simulink library "inp"  (R2021b)
settings: Solver=VariableStepAuto  StartTime=0.0  StopTime=10.0  RelTol=1e-3
undefined symbols (not defined in the file): C_TASK_5MS_S, FALSE, KINP_AcoreReadyToSlp_flg_ovrdflg, KINP_AcoreReadyToSlp_flg_ovrdval, KINP_AllowMovThd_OTA_enum_ovrdflg, KINP_AllowMovThd_OTA_enum_ovrdval, KINP_APSAngleTarget_Deg_ovrdflg, KINP_APSAngleTarget_Deg_ovrdval, KINP_APSDecReq_mps2_ovrdflg, KINP_APSDecReq_mps2_ovrdval, KINP_APSDecReqA_flg_ovrdflg, KINP_APSDecReqA_flg_ovrdval, KINP_APSDFLL_cm_ovrdflg, KINP_APSDFLL_cm_ovrdval, KINP_APSDFLR_cm_ovrdflg, KINP_APSDFLR_cm_ovrdval, KINP_APSDRLL_cm_ovrdflg, KINP_APSDRLL_cm_ovrdval, KINP_APSDRLR_cm_ovrdflg, KINP_APSDRLR_cm_ovrdval, KINP_APSExitCondition_enum_ovrdflg, KINP_APSExitCondition_enum_ovrdval, KINP_APSHWVer_enum_ovrdflg, KINP_APSHWVer_enum_ovrdval, KINP_APSProgressPCT_pct_ovrdflg, KINP_APSProgressPCT_pct_ovrdval, KINP_APSPwrReq_enum_ovrdflg, KINP_APSPwrReq_enum_ovrdval, KINP_APSReq_enum_ovrdflg, KINP_APSReq_enum_ovrdval, KINP_APSRQDisplay_enum_ovrdflg, KINP_APSRQDisplay_enum_ovrdval, KINP_APSRqEPASCtrl_flg_ovrdflg, KINP_APSRqEPASCtrl_flg_ovrdval, KINP_APSShiftPosnReq_enum_ovrdval, KINP_APSShiftPosnReq_enum_ovrflg, KINP_APSSpeedCMD_kph_ovrdval, KINP_APSSpeedCMD_kph_ovrflg, KINP_APSStaSystem_enum_ovrdflg, KINP_APSStaSystem_enum_ovrdval, KINP_APSSWVer_enum_ovrdflg, KINP_APSSWVer_enum_ovrdval, KINP_APSVMCReqA_flg_ovrdval, KINP_APSVMCReqA_flg_ovrflg, KINP_APSVRqEPASCtrl_flg_ovrdflg, KINP_APSVRqEPASCtrl_flg_ovrdval, KINP_AuxBattVolmV_mV_ovrdflg, KINP_AuxBattVolmV_mV_ovrdval, KINP_BTConnectSta_enum_ovrdflg, KINP_BTConnectSta_enum_ovrdval, KINP_CAASSta_enum_ovrdflg, KINP_CAASSta_enum_ovrdval, KINP_CAASVMCReqA_flg_ovrdval, KINP_CAASVMCReqA_flg_ovrflg, KINP_CAN1BusOff_flg_ovrdflg, KINP_CAN1BusOff_flg_ovrdval, KINP_CAN2BusOff_flg_ovrdflg, KINP_CAN2BusOff_flg_ovrdval, KINP_CAN3BusOff_flg_ovrdflg, KINP_CAN3BusOff_flg_ovrdval ... (+222)
libraries: FVT_lib x1035, hcu_lib x1
(part 24 of 33)

== system inp/INP/CAN3/SignalCheck/MCU_N_F2 ==
  BHAL_outputs : Inport
  inp_CanValid_bus : Inport  Port=2
  FrCoolanttempReqNidec : FVT_lib/inp/can_signal_template  SystemSampleTime=-1  VariantActivationTime=update diagram  Latency=0  AutoFrameSizeCalculation=off
      link override defval: Value=KINP_FrCoolanttempReqNidec_C_defval
      link override ovrdflg: Value=KINP_FrCoolanttempReqNidec_C_ovrdflg
      link override ovrdval: Value=KINP_FrCoolanttempReqNidec_C_ovrdval
  FrEOPSpdSetNidec : FVT_lib/inp/can_signal_template  SystemSampleTime=-1  VariantActivationTime=update diagram  Latency=0  AutoFrameSizeCalculation=off
      link override defval: Value=KINP_FrEOPSpdSetNidec_rpm_defval
      link override ovrdflg: Value=KINP_FrEOPSpdSetNidec_rpm_ovrdflg
      link override ovrdval: Value=KINP_FrEOPSpdSetNidec_rpm_ovrdval
  FrFailcode1Nidec : FVT_lib/inp/can_signal_template  SystemSampleTime=-1  VariantActivationTime=update diagram  Latency=0  AutoFrameSizeCalculation=off
      link override defval: Value=KINP_FrFailcode1Nidec_enum_defval
      link override ovrdflg: Value=KINP_FrFailcode1Nidec_enum_ovrdflg
      link override ovrdval: Value=KINP_FrFailcode1Nidec_enum_ovrdval
  FrFailcode2Nidec : FVT_lib/inp/can_signal_template  SystemSampleTime=-1  VariantActivationTime=update diagram  Latency=0  AutoFrameSizeCalculation=off
      link override defval: Value=KINP_FrFailcode2Nidec_enum_defval
      link override ovrdflg: Value=KINP_FrFailcode2Nidec_enum_ovrdflg
      link override ovrdval: Value=KINP_FrFailcode2Nidec_enum_ovrdval
  FrFailcodehistory1Nidec : FVT_lib/inp/can_signal_template  SystemSampleTime=-1  VariantActivationTime=update diagram  Latency=0  AutoFrameSizeCalculation=off
      link override defval: Value=KINP_FrFailcodehistory1Nidec_enum_defval
      link override ovrdflg: Value=KINP_FrFailcodehistory1Nidec_enum_ovrdflg
      link override ovrdval: Value=KINP_FrFailcodehistory1Nidec_enum_ovrdval
  FrFailcodehistory2Nidec : FVT_lib/inp/can_signal_template  SystemSampleTime=-1  VariantActivationTime=update diagram  Latency=0  AutoFrameSizeCalculation=off
      link override defval: Value=KINP_FrFailcodehistory2Nidec_enum_defval
      link override ovrdflg: Value=KINP_FrFailcodehistory2Nidec_enum_ovrdflg
      link override ovrdval: Value=KINP_FrFailcodehistory2Nidec_enum_ovrdval
  FrLLCTempNidec : FVT_lib/inp/can_signal_template  SystemSampleTime=-1  VariantActivationTime=update diagram  Latency=0  AutoFrameSizeCalculation=off
      link override defval: Value=KINP_FrLLCTempNidec_C_defval
      link override ovrdflg: Value=KINP_FrLLCTempNidec_C_ovrdflg
      link override ovrdval: Value=KINP_FrLLCTempNidec_C_ovrdval
  FrLLCflowReqNidec : FVT_lib/inp/can_signal_template  SystemSampleTime=-1  VariantActivationTime=update diagram  Latency=0  AutoFrameSizeCalculation=off
      link override defval: Value=KINP_FrLLCflowReqNidec_Lpmin_defval
      link override ovrdflg: Value=KINP_FrLLCflowReqNidec_Lpmin_ovrdflg
      link override ovrdval: Value=KINP_FrLLCflowReqNidec_Lpmin_ovrdval
  FrMCUTempWarnNidec : FVT_lib/inp/can_signal_template  SystemSampleTime=-1  VariantActivationTime=update diagram  Latency=0  AutoFrameSizeCalculation=off
      link override defval: Value=KINP_FrMCUTempWarnNidec_enum_defval
      link override ovrdflg: Value=KINP_FrMCUTempWarnNidec_enum_ovrdflg
      link override ovrdval: Value=KINP_FrMCUTempWarnNidec_enum_ovrdval
  FrTMTempWarnNidec : FVT_lib/inp/can_signal_template  SystemSampleTime=-1  VariantActivationTime=update diagram  Latency=0  AutoFrameSizeCalculation=off
      link override defval: Value=KINP_FrTMTempWarnNidec_enum_defval
      link override ovrdflg: Value=KINP_FrTMTempWarnNidec_enum_ovrdflg
      link override ovrdval: Value=KINP_FrTMTempWarnNidec_enum_ovrdval
  Terminator_{1..10} (10 alike) : Terminator
  True_VHAL_FrCoolanttempReqNidec_C : Constant  Value=TRUE  OutDataTypeStr=boolean
  True_VHAL_FrEOPSpdSetNidec_rpm : Constant  Value=TRUE  OutDataTypeStr=boolean
  True_VHAL_FrFailcode1Nidec_enum : Constant  Value=TRUE  OutDataTypeStr=boolean
  True_VHAL_FrFailcode2Nidec_enum : Constant  Value=TRUE  OutDataTypeStr=boolean
  True_VHAL_FrFailcodehistory1Nidec_enum : Constant  Value=TRUE  OutDataTypeStr=boolean
  True_VHAL_FrFailcodehistory2Nidec_enum : Constant  Value=TRUE  OutDataTypeStr=boolean
  True_VHAL_FrLLCTempNidec_C : Constant  Value=TRUE  OutDataTypeStr=boolean
  True_VHAL_FrLLCflowReqNidec_Lpmin : Constant  Value=TRUE  OutDataTypeStr=boolean
  True_VHAL_FrMCUTempWarnNidec_enum : Constant  Value=TRUE  OutDataTypeStr=boolean
  True_VHAL_FrTMTempWarnNidec_enum : Constant  Value=TRUE  OutDataTypeStr=boolean
  slr1_{1..10} (10 alike) : BusSelector  OutputSignals=VINP_CANMsgValidMCUNF2_flg
  slr_VHAL_FrCoolanttempReqNidec_C : BusSelector  OutputSignals=VHAL_FrCoolanttempReqNidec_C
  slr_VHAL_FrEOPSpdSetNidec_rpm : BusSelector  OutputSignals=VHAL_FrEOPSpdSetNidec_rpm
  slr_VHAL_FrFailcode1Nidec_enum : BusSelector  OutputSignals=VHAL_FrFailcode1Nidec_enum
  slr_VHAL_FrFailcode2Nidec_enum : BusSelector  OutputSignals=VHAL_FrFailcode2Nidec_enum
  slr_VHAL_FrFailcodehistory1Nidec_enum : BusSelector  OutputSignals=VHAL_FrFailcodehistory1Nidec_enum
  slr_VHAL_FrFailcodehistory2Nidec_enum : BusSelector  OutputSignals=VHAL_FrFailcodehistory2Nidec_enum
  slr_VHAL_FrLLCTempNidec_C : BusSelector  OutputSignals=VHAL_FrLLCTempNidec_C
  slr_VHAL_FrLLCflowReqNidec_Lpmin : BusSelector  OutputSignals=VHAL_FrLLCflowReqNidec_Lpmin
  slr_VHAL_FrMCUTempWarnNidec_enum : BusSelector  OutputSignals=VHAL_FrMCUTempWarnNidec_enum
  slr_VHAL_FrTMTempWarnNidec_enum : BusSelector  OutputSignals=VHAL_FrTMTempWarnNidec_enum
  VINP_FrCoolanttempReqNidec_C : Outport
  VINP_FrEOPSpdSetNidec_rpm : Outport  Port=2
  VINP_FrFailcode1Nidec_enum : Outport  Port=3
  VINP_FrFailcode2Nidec_enum : Outport  Port=4
  VINP_FrFailcodehistory1Nidec_enum : Outport  Port=5
  VINP_FrFailcodehistory2Nidec_enum : Outport  Port=6
  VINP_FrLLCTempNidec_C : Outport  Port=7
  VINP_FrLLCflowReqNidec_Lpmin : Outport  Port=8
  VINP_FrMCUTempWarnNidec_enum : Outport  Port=9
  VINP_FrTMTempWarnNidec_enum : Outport  Port=10
  wires:
  BHAL_outputs/1 -> [BHAL_outputs]
  inp_CanValid_bus/1 -> [inp_CanValid_bus]
  [BHAL_outputs] -> slr_VHAL_FrCoolanttempReqNidec_C/1
  slr_VHAL_FrCoolanttempReqNidec_C/1 -> FrCoolanttempReqNidec/1  "<VHAL_FrCoolanttempReqNidec_C>"
  True_VHAL_FrCoolanttempReqNidec_C/1 -> FrCoolanttempReqNidec/2
  [inp_CanValid_bus] -> slr1_1/1
  slr1_1/1 -> FrCoolanttempReqNidec/3  "<VINP_CANMsgValidMCUNF2_flg>"
  FrCoolanttempReqNidec/1 -> VINP_FrCoolanttempReqNidec_C/1  "VINP_FrCoolanttempReqNidec_C"
  FrCoolanttempReqNidec/2 -> Terminator_1/1
  [BHAL_outputs] -> slr_VHAL_FrEOPSpdSetNidec_rpm/1
  slr_VHAL_FrEOPSpdSetNidec_rpm/1 -> FrEOPSpdSetNidec/1  "<VHAL_FrEOPSpdSetNidec_rpm>"
  True_VHAL_FrEOPSpdSetNidec_rpm/1 -> FrEOPSpdSetNidec/2
  [inp_CanValid_bus] -> slr1_2/1
  slr1_2/1 -> FrEOPSpdSetNidec/3  "<VINP_CANMsgValidMCUNF2_flg>"
  FrEOPSpdSetNidec/1 -> VINP_FrEOPSpdSetNidec_rpm/1  "VINP_FrEOPSpdSetNidec_rpm"
  FrEOPSpdSetNidec/2 -> Terminator_2/1
  [BHAL_outputs] -> slr_VHAL_FrFailcode1Nidec_enum/1
  slr_VHAL_FrFailcode1Nidec_enum/1 -> FrFailcode1Nidec/1  "<VHAL_FrFailcode1Nidec_enum>"
  True_VHAL_FrFailcode1Nidec_enum/1 -> FrFailcode1Nidec/2
  [inp_CanValid_bus] -> slr1_3/1
  slr1_3/1 -> FrFailcode1Nidec/3  "<VINP_CANMsgValidMCUNF2_flg>"
  FrFailcode1Nidec/1 -> VINP_FrFailcode1Nidec_enum/1  "VINP_FrFailcode1Nidec_enum"
  FrFailcode1Nidec/2 -> Terminator_3/1
  [BHAL_outputs] -> slr_VHAL_FrFailcode2Nidec_enum/1
  slr_VHAL_FrFailcode2Nidec_enum/1 -> FrFailcode2Nidec/1  "<VHAL_FrFailcode2Nidec_enum>"
  True_VHAL_FrFailcode2Nidec_enum/1 -> FrFailcode2Nidec/2
  [inp_CanValid_bus] -> slr1_4/1
  slr1_4/1 -> FrFailcode2Nidec/3  "<VINP_CANMsgValidMCUNF2_flg>"
  FrFailcode2Nidec/1 -> VINP_FrFailcode2Nidec_enum/1  "VINP_FrFailcode2Nidec_enum"
  FrFailcode2Nidec/2 -> Terminator_4/1
  [BHAL_outputs] -> slr_VHAL_FrFailcodehistory1Nidec_enum/1
  slr_VHAL_FrFailcodehistory1Nidec_enum/1 -> FrFailcodehistory1Nidec/1  "<VHAL_FrFailcodehistory1Nidec_enum>"
  True_VHAL_FrFailcodehistory1Nidec_enum/1 -> FrFailcodehistory1Nidec/2
  [inp_CanValid_bus] -> slr1_5/1
  slr1_5/1 -> FrFailcodehistory1Nidec/3  "<VINP_CANMsgValidMCUNF2_flg>"
  FrFailcodehistory1Nidec/1 -> VINP_FrFailcodehistory1Nidec_enum/1  "VINP_FrFailcodehistory1Nidec_enum"
  FrFailcodehistory1Nidec/2 -> Terminator_5/1
  [BHAL_outputs] -> slr_VHAL_FrFailcodehistory2Nidec_enum/1
  slr_VHAL_FrFailcodehistory2Nidec_enum/1 -> FrFailcodehistory2Nidec/1  "<VHAL_FrFailcodehistory2Nidec_enum>"
  True_VHAL_FrFailcodehistory2Nidec_enum/1 -> FrFailcodehistory2Nidec/2
  [inp_CanValid_bus] -> slr1_6/1
  slr1_6/1 -> FrFailcodehistory2Nidec/3  "<VINP_CANMsgValidMCUNF2_flg>"
  FrFailcodehistory2Nidec/1 -> VINP_FrFailcodehistory2Nidec_enum/1  "VINP_FrFailcodehistory2Nidec_enum"
  FrFailcodehistory2Nidec/2 -> Terminator_6/1
  [BHAL_outputs] -> slr_VHAL_FrLLCTempNidec_C/1
  slr_VHAL_FrLLCTempNidec_C/1 -> FrLLCTempNidec/1  "<VHAL_FrLLCTempNidec_C>"
  True_VHAL_FrLLCTempNidec_C/1 -> FrLLCTempNidec/2
  [inp_CanValid_bus] -> slr1_7/1
  slr1_7/1 -> FrLLCTempNidec/3  "<VINP_CANMsgValidMCUNF2_flg>"
  FrLLCTempNidec/1 -> VINP_FrLLCTempNidec_C/1  "VINP_FrLLCTempNidec_C"
  FrLLCTempNidec/2 -> Terminator_7/1
  [BHAL_outputs] -> slr_VHAL_FrLLCflowReqNidec_Lpmin/1
  slr_VHAL_FrLLCflowReqNidec_Lpmin/1 -> FrLLCflowReqNidec/1  "<VHAL_FrLLCflowReqNidec_Lpmin>"
  True_VHAL_FrLLCflowReqNidec_Lpmin/1 -> FrLLCflowReqNidec/2
  [inp_CanValid_bus] -> slr1_8/1
  slr1_8/1 -> FrLLCflowReqNidec/3  "<VINP_CANMsgValidMCUNF2_flg>"
  FrLLCflowReqNidec/1 -> VINP_FrLLCflowReqNidec_Lpmin/1  "VINP_FrLLCflowReqNidec_Lpmin"
  FrLLCflowReqNidec/2 -> Terminator_8/1
  [BHAL_outputs] -> slr_VHAL_FrMCUTempWarnNidec_enum/1
  slr_VHAL_FrMCUTempWarnNidec_enum/1 -> FrMCUTempWarnNidec/1  "<VHAL_FrMCUTempWarnNidec_enum>"
  True_VHAL_FrMCUTempWarnNidec_enum/1 -> FrMCUTempWarnNidec/2
  [inp_CanValid_bus] -> slr1_9/1
  slr1_9/1 -> FrMCUTempWarnNidec/3  "<VINP_CANMsgValidMCUNF2_flg>"
  FrMCUTempWarnNidec/1 -> VINP_FrMCUTempWarnNidec_enum/1  "VINP_FrMCUTempWarnNidec_enum"
  FrMCUTempWarnNidec/2 -> Terminator_9/1
  [BHAL_outputs] -> slr_VHAL_FrTMTempWarnNidec_enum/1
  slr_VHAL_FrTMTempWarnNidec_enum/1 -> FrTMTempWarnNidec/1  "<VHAL_FrTMTempWarnNidec_enum>"
  True_VHAL_FrTMTempWarnNidec_enum/1 -> FrTMTempWarnNidec/2
  [inp_CanValid_bus] -> slr1_10/1
  slr1_10/1 -> FrTMTempWarnNidec/3  "<VINP_CANMsgValidMCUNF2_flg>"
  FrTMTempWarnNidec/1 -> VINP_FrTMTempWarnNidec_enum/1  "VINP_FrTMTempWarnNidec_enum"
  FrTMTempWarnNidec/2 -> Terminator_10/1

== system inp/INP/CAN3/SignalCheck/MCU_N_F3 ==
  BHAL_outputs : Inport
  inp_CanValid_bus : Inport  Port=2
  FrMCUHWVerNidec : FVT_lib/inp/can_signal_template  SystemSampleTime=-1  VariantActivationTime=update diagram  Latency=0  AutoFrameSizeCalculation=off
      link override defval: Value=KINP_FrMCUHWVerNidec_enum_defval
      link override ovrdflg: Value=KINP_FrMCUHWVerNidec_enum_ovrdflg
      link override ovrdval: Value=KINP_FrMCUHWVerNidec_enum_ovrdval
  FrMCUSWVerNidec : FVT_lib/inp/can_signal_template  SystemSampleTime=-1  VariantActivationTime=update diagram  Latency=0  AutoFrameSizeCalculation=off
      link override defval: Value=KINP_FrMCUSWVerNidec_enum_defval
      link override ovrdflg: Value=KINP_FrMCUSWVerNidec_enum_ovrdflg
      link override ovrdval: Value=KINP_FrMCUSWVerNidec_enum_ovrdval
  Terminator_1 : Terminator
  Terminator_2 : Terminator
  True_VHAL_FrMCUHWVerNidec_enum : Constant  Value=TRUE  OutDataTypeStr=boolean
  True_VHAL_FrMCUSWVerNidec_enum : Constant  Value=TRUE  OutDataTypeStr=boolean
  slr1_1 : BusSelector  OutputSignals=VINP_CANMsgValidMCUNF3_flg
  slr1_2 : BusSelector  OutputSignals=VINP_CANMsgValidMCUNF3_flg
  slr_VHAL_FrMCUHWVerNidec_enum : BusSelector  OutputSignals=VHAL_FrMCUHWVerNidec_enum
  slr_VHAL_FrMCUSWVerNidec_enum : BusSelector  OutputSignals=VHAL_FrMCUSWVerNidec_enum
  VINP_FrMCUHWVerNidec_enum : Outport
  VINP_FrMCUSWVerNidec_enum : Outport  Port=2
  wires:
  BHAL_outputs/1 -> [BHAL_outputs]
  inp_CanValid_bus/1 -> [inp_CanValid_bus]
  [BHAL_outputs] -> slr_VHAL_FrMCUHWVerNidec_enum/1
  slr_VHAL_FrMCUHWVerNidec_enum/1 -> FrMCUHWVerNidec/1  "<VHAL_FrMCUHWVerNidec_enum>"
  True_VHAL_FrMCUHWVerNidec_enum/1 -> FrMCUHWVerNidec/2
  [inp_CanValid_bus] -> slr1_1/1
  slr1_1/1 -> FrMCUHWVerNidec/3  "<VINP_CANMsgValidMCUNF3_flg>"
  FrMCUHWVerNidec/1 -> VINP_FrMCUHWVerNidec_enum/1  "VINP_FrMCUHWVerNidec_enum"
  FrMCUHWVerNidec/2 -> Terminator_1/1
  [BHAL_outputs] -> slr_VHAL_FrMCUSWVerNidec_enum/1
  slr_VHAL_FrMCUSWVerNidec_enum/1 -> FrMCUSWVerNidec/1  "<VHAL_FrMCUSWVerNidec_enum>"
  True_VHAL_FrMCUSWVerNidec_enum/1 -> FrMCUSWVerNidec/2
  [inp_CanValid_bus] -> slr1_2/1
  slr1_2/1 -> FrMCUSWVerNidec/3  "<VINP_CANMsgValidMCUNF3_flg>"
  FrMCUSWVerNidec/1 -> VINP_FrMCUSWVerNidec_enum/1  "VINP_FrMCUSWVerNidec_enum"
  FrMCUSWVerNidec/2 -> Terminator_2/1

== system inp/INP/CAN3/SignalCheck/MCU_N_R1 ==
  BHAL_outputs : Inport
  inp_CanValid_bus : Inport  Port=2
  MCUNR1CSErr : FVT_lib/inp/can_signal_template  SystemSampleTime=-1  VariantActivationTime=update diagram  Latency=0  AutoFrameSizeCalculation=off
      link override defval: Value=KINP_MCUNR1CSErr_flg_defval
      link override ovrdflg: Value=KINP_MCUNR1CSErr_flg_ovrdflg
      link override ovrdval: Value=KINP_MCUNR1CSErr_flg_ovrdval
  MCUNR1RCErr : FVT_lib/inp/can_signal_template  SystemSampleTime=-1  VariantActivationTime=update diagram  Latency=0  AutoFrameSizeCalculation=off
      link override defval: Value=KINP_MCUNR1RCErr_flg_defval
      link override ovrdflg: Value=KINP_MCUNR1RCErr_flg_ovrdflg
      link override ovrdval: Value=KINP_MCUNR1RCErr_flg_ovrdval
  MCUWarnRNidec : FVT_lib/inp/can_signal_template  SystemSampleTime=-1  VariantActivationTime=update diagram  Latency=0  AutoFrameSizeCalculation=off
      link override defval: Value=KINP_MCUWarnRNidec_enum_defval
      link override ovrdflg: Value=KINP_MCUWarnRNidec_enum_ovrdflg
      link override ovrdval: Value=KINP_MCUWarnRNidec_enum_ovrdval
  RrActvDmpDisabStaNidec : FVT_lib/inp/can_signal_template  SystemSampleTime=-1  VariantActivationTime=update diagram  Latency=0  AutoFrameSizeCalculation=off
      link override defval: Value=KINP_RrActvDmpDisabStaNidec_flg_defval
      link override ovrdflg: Value=KINP_RrActvDmpDisabStaNidec_flg_ovrdflg
      link override ovrdval: Value=KINP_RrActvDmpDisabStaNidec_flg_ovrdval
  RrEDUDrtStaNidec : FVT_lib/inp/can_signal_template  SystemSampleTime=-1  VariantActivationTime=update diagram  Latency=0  AutoFrameSizeCalculation=off
      link override defval: Value=KINP_RrEDUDrtStaNidec_flg_defval
      link override ovrdflg: Value=KINP_RrEDUDrtStaNidec_flg_ovrdflg
      link override ovrdval: Value=KINP_RrEDUDrtStaNidec_flg_ovrdval
  RrEDUOpratingStaNidec : FVT_lib/inp/can_signal_template  SystemSampleTime=-1  VariantActivationTime=update diagram  Latency=0  AutoFrameSizeCalculation=off
      link override defval: Value=KINP_RrEDUOpratingStaNidec_flg_defval
      link override ovrdflg: Value=KINP_RrEDUOpratingStaNidec_flg_ovrdflg
      link override ovrdval: Value=KINP_RrEDUOpratingStaNidec_flg_ovrdval
  RrEDURealTMTqNidec : FVT_lib/inp/can_signal_template  SystemSampleTime=-1  VariantActivationTime=update diagram  Latency=0  AutoFrameSizeCalculation=off
      link override defval: Value=KINP_RrEDURealTMTqNidec_Nm_defval
      link override ovrdflg: Value=KINP_RrEDURealTMTqNidec_Nm_ovrdflg
      link override ovrdval: Value=KINP_RrEDURealTMTqNidec_Nm_ovrdval
  RrEDURotateDirctionNidec : FVT_lib/inp/can_signal_template  SystemSampleTime=-1  VariantActivationTime=update diagram  Latency=0  AutoFrameSizeCalculation=off
      link override defval: Value=KINP_RrEDURotateDirctionNidec_enum_defval
      link override ovrdflg: Value=KINP_RrEDURotateDirctionNidec_enum_ovrdflg
      link override ovrdval: Value=KINP_RrEDURotateDirctionNidec_enum_ovrdval
  RrEDUTqReqFbkNidec : FVT_lib/inp/can_signal_template  SystemSampleTime=-1  VariantActivationTime=update diagram  Latency=0  AutoFrameSizeCalculation=off
      link override defval: Value=KINP_RrEDUTqReqFbkNidec_Nm_defval
      link override ovrdflg: Value=KINP_RrEDUTqReqFbkNidec_Nm_ovrdflg
      link override ovrdval: Value=KINP_RrEDUTqReqFbkNidec_Nm_ovrdval
  RrMCU1ChksumNidec : FVT_lib/inp/can_signal_template  SystemSampleTime=-1  VariantActivationTime=update diagram  Latency=0  AutoFrameSizeCalculation=off
      link override defval: Value=KINP_RrMCU1ChksumNidec_enum_defval
      link override ovrdflg: Value=KINP_RrMCU1ChksumNidec_enum_ovrdflg
      link override ovrdval: Value=KINP_RrMCU1ChksumNidec_enum_ovrdval
  RrMCU1RolCntNidec : FVT_lib/inp/can_signal_template  SystemSampleTime=-1  VariantActivationTime=update diagram  Latency=0  AutoFrameSizeCalculation=off
      link override defval: Value=KINP_RrMCU1RolCntNidec_enum_defval
      link override ovrdflg: Value=KINP_RrMCU1RolCntNidec_enum_ovrdflg
      link override ovrdval: Value=KINP_RrMCU1RolCntNidec_enum_ovrdval
  RrMCUBATNidec : FVT_lib/inp/can_signal_template  SystemSampleTime=-1  VariantActivationTime=update diagram  Latency=0  AutoFrameSizeCalculation=off
      link override defval: Value=KINP_RrMCUBATNidec_V_defval
      link override ovrdflg: Value=KINP_RrMCUBATNidec_V_ovrdflg
      link override ovrdval: Value=KINP_RrMCUBATNidec_V_ovrdval
  RrMCUDCBusCurrNidec : FVT_lib/inp/can_signal_template  SystemSampleTime=-1  VariantActivationTime=update diagram  Latency=0  AutoFrameSizeCalculation=off
      link override defval: Value=KINP_RrMCUDCBusCurrNidec_A_defval
      link override ovrdflg: Value=KINP_RrMCUDCBusCurrNidec_A_ovrdflg
      link override ovrdval: Value=KINP_RrMCUDCBusCurrNidec_A_ovrdval
  RrMCUDCBusVoltNidec : FVT_lib/inp/can_signal_template  SystemSampleTime=-1  VariantActivationTime=update diagram  Latency=0  AutoFrameSizeCalculation=off
      link override defval: Value=KINP_RrMCUDCBusVoltNidec_V_defval
      link override ovrdflg: Value=KINP_RrMCUDCBusVoltNidec_V_ovrdflg
      link override ovrdval: Value=KINP_RrMCUDCBusVoltNidec_V_ovrdval
  RrMCUDischrgStaNidec : FVT_lib/inp/can_signal_template  SystemSampleTime=-1  VariantActivationTime=update diagram  Latency=0  AutoFrameSizeCalculation=off
      link override defval: Value=KINP_RrMCUDischrgStaNidec_flg_defval
      link override ovrdflg: Value=KINP_RrMCUDischrgStaNidec_flg_ovrdflg
      link override ovrdval: Value=KINP_RrMCUDischrgStaNidec_flg_ovrdval
  RrMCUEnaStaNidec : FVT_lib/inp/can_signal_template  SystemSampleTime=-1  VariantActivationTime=update diagram  Latency=0  AutoFrameSizeCalculation=off
      link override defval: Value=KINP_RrMCUEnaStaNidec_flg_defval
      link override ovrdflg: Value=KINP_RrMCUEnaStaNidec_flg_ovrdflg
      link override ovrdval: Value=KINP_RrMCUEnaStaNidec_flg_ovrdval
  RrMCUErrNidec : FVT_lib/inp/can_signal_template  SystemSampleTime=-1  VariantActivationTime=update diagram  Latency=0  AutoFrameSizeCalculation=off
      link override defval: Value=KINP_RrMCUErrNidec_enum_defval
      link override ovrdflg: Value=KINP_RrMCUErrNidec_enum_ovrdflg
      link override ovrdval: Value=KINP_RrMCUErrNidec_enum_ovrdval
  RrMCUIGNstaNidec : FVT_lib/inp/can_signal_template  SystemSampleTime=-1  VariantActivationTime=update diagram  Latency=0  AutoFrameSizeCalculation=off
      link override defval: Value=KINP_RrMCUIGNstaNidec_flg_defval
      link override ovrdflg: Value=KINP_RrMCUIGNstaNidec_flg_ovrdflg
      link override ovrdval: Value=KINP_RrMCUIGNstaNidec_flg_ovrdval
  RrMCUReady4PreNidec : FVT_lib/inp/can_signal_template  SystemSampleTime=-1  VariantActivationTime=update diagram  Latency=0  AutoFrameSizeCalculation=off
      link override defval: Value=KINP_RrMCUReady4PreNidec_flg_defval
      link override ovrdflg: Value=KINP_RrMCUReady4PreNidec_flg_ovrdflg
      link override ovrdval: Value=KINP_RrMCUReady4PreNidec_flg_ovrdval
  RrMCUReadyNidec : FVT_lib/inp/can_signal_template  SystemSampleTime=-1  VariantActivationTime=update diagram  Latency=0  AutoFrameSizeCalculation=off
      link override defval: Value=KINP_RrMCUReadyNidec_flg_defval
      link override ovrdflg: Value=KINP_RrMCUReadyNidec_flg_ovrdflg
      link override ovrdval: Value=KINP_RrMCUReadyNidec_flg_ovrdval
  RrMCUSysStaNidec : FVT_lib/inp/can_signal_template  SystemSampleTime=-1  VariantActivationTime=update diagram  Latency=0  AutoFrameSizeCalculation=off
      link override defval: Value=KINP_RrMCUSysStaNidec_enum_defval
      link override ovrdflg: Value=KINP_RrMCUSysStaNidec_enum_ovrdflg
      link override ovrdval: Value=KINP_RrMCUSysStaNidec_enum_ovrdval
  RrMCUTempNidec : FVT_lib/inp/can_signal_template  SystemSampleTime=-1  VariantActivationTime=update diagram  Latency=0  AutoFrameSizeCalculation=off
      link override defval: Value=KINP_RrMCUTempNidec_C_defval
      link override ovrdflg: Value=KINP_RrMCUTempNidec_C_ovrdflg
      link override ovrdval: Value=KINP_RrMCUTempNidec_C_ovrdval
  RrMotorAvailTqNidec : FVT_lib/inp/can_signal_template  SystemSampleTime=-1  VariantActivationTime=update diagram  Latency=0  AutoFrameSizeCalculation=off
      link override defval: Value=KINP_RrMotorAvailTqNidec_Nm_defval
      link override ovrdflg: Value=KINP_RrMotorAvailTqNidec_Nm_ovrdflg
      link override ovrdval: Value=KINP_RrMotorAvailTqNidec_Nm_ovrdval
  RrRegenAvailTqNidec : FVT_lib/inp/can_signal_template  SystemSampleTime=-1  VariantActivationTime=update diagram  Latency=0  AutoFrameSizeCalculation=off
      link override defval: Value=KINP_RrRegenAvailTqNidec_Nm_defval
      link override ovrdflg: Value=KINP_RrRegenAvailTqNidec_Nm_ovrdflg
      link override ovrdval: Value=KINP_RrRegenAvailTqNidec_Nm_ovrdval
  RrTMSpdNidec : FVT_lib/inp/can_signal_template  SystemSampleTime=-1  VariantActivationTime=update diagram  Latency=0  AutoFrameSizeCalculation=off
      link override defval: Value=KINP_RrTMSpdNidec_rpm_defval
      link override ovrdflg: Value=KINP_RrTMSpdNidec_rpm_ovrdflg
      link override ovrdval: Value=KINP_RrTMSpdNidec_rpm_ovrdval
  RrTMTempNidec : FVT_lib/inp/can_signal_template  SystemSampleTime=-1  VariantActivationTime=update diagram  Latency=0  AutoFrameSizeCalculation=off
      link override defval: Value=KINP_RrTMTempNidec_C_defval
      link override ovrdflg: Value=KINP_RrTMTempNidec_C_ovrdflg
      link override ovrdval: Value=KINP_RrTMTempNidec_C_ovrdval
  RrTMidNidec : FVT_lib/inp/can_signal_template  SystemSampleTime=-1  VariantActivationTime=update diagram  Latency=0  AutoFrameSizeCalculation=off
      link override defval: Value=KINP_RrTMidNidec_A_defval
      link override ovrdflg: Value=KINP_RrTMidNidec_A_ovrdflg
      link override ovrdval: Value=KINP_RrTMidNidec_A_ovrdval
  RrTMiqNidec : FVT_lib/inp/can_signal_template  SystemSampleTime=-1  VariantActivationTime=update diagram  Latency=0  AutoFrameSizeCalculation=off
      link override defval: Value=KINP_RrTMiqNidec_A_defval
      link override ovrdflg: Value=KINP_RrTMiqNidec_A_ovrdflg
      link override ovrdval: Value=KINP_RrTMiqNidec_A_ovrdval
  Terminator_{1..28} (28 alike) : Terminator
  True_VHAL_MCUNR1CSErr_flg : Constant  Value=TRUE  OutDataTypeStr=boolean
  True_VHAL_MCUNR1RCErr_flg : Constant  Value=TRUE  OutDataTypeStr=boolean
  True_VHAL_MCUWarnRNidec_enum : Constant  Value=TRUE  OutDataTypeStr=boolean
  True_VHAL_RrActvDmpDisabStaNidec_flg : Constant  Value=TRUE  OutDataTypeStr=boolean
  True_VHAL_RrEDUDrtStaNidec_flg : Constant  Value=TRUE  OutDataTypeStr=boolean
  True_VHAL_RrEDUOpratingStaNidec_flg : Constant  Value=TRUE  OutDataTypeStr=boolean
  True_VHAL_RrEDURealTMTqNidec_Nm : Constant  Value=TRUE  OutDataTypeStr=boolean
  True_VHAL_RrEDURotateDirctionNidec_enum : Constant  Value=TRUE  OutDataTypeStr=boolean
  True_VHAL_RrEDUTqReqFbkNidec_Nm : Constant  Value=TRUE  OutDataTypeStr=boolean
  True_VHAL_RrMCU1ChksumNidec_enum : Constant  Value=TRUE  OutDataTypeStr=boolean
  True_VHAL_RrMCU1RolCntNidec_enum : Constant  Value=TRUE  OutDataTypeStr=boolean
  True_VHAL_RrMCUBATNidec_V : Constant  Value=TRUE  OutDataTypeStr=boolean
  True_VHAL_RrMCUDCBusCurrNidec_A : Constant  Value=TRUE  OutDataTypeStr=boolean
  True_VHAL_RrMCUDCBusVoltNidec_V : Constant  Value=TRUE  OutDataTypeStr=boolean
  True_VHAL_RrMCUDischrgStaNidec_flg : Constant  Value=TRUE  OutDataTypeStr=boolean
  True_VHAL_RrMCUEnaStaNidec_flg : Constant  Value=TRUE  OutDataTypeStr=boolean
  True_VHAL_RrMCUErrNidec_enum : Constant  Value=TRUE  OutDataTypeStr=boolean
  True_VHAL_RrMCUIGNstaNidec_flg : Constant  Value=TRUE  OutDataTypeStr=boolean
  True_VHAL_RrMCUReady4PreNidec_flg : Constant  Value=TRUE  OutDataTypeStr=boolean
  True_VHAL_RrMCUReadyNidec_flg : Constant  Value=TRUE  OutDataTypeStr=boolean
  True_VHAL_RrMCUSysStaNidec_enum : Constant  Value=TRUE  OutDataTypeStr=boolean
  True_VHAL_RrMCUTempNidec_C : Constant  Value=TRUE  OutDataTypeStr=boolean
  True_VHAL_RrMotorAvailTqNidec_Nm : Constant  Value=TRUE  OutDataTypeStr=boolean
  True_VHAL_RrRegenAvailTqNidec_Nm : Constant  Value=TRUE  OutDataTypeStr=boolean
  True_VHAL_RrTMSpdNidec_rpm : Constant  Value=TRUE  OutDataTypeStr=boolean
  True_VHAL_RrTMTempNidec_C : Constant  Value=TRUE  OutDataTypeStr=boolean
  True_VHAL_RrTMidNidec_A : Constant  Value=TRUE  OutDataTypeStr=boolean
  True_VHAL_RrTMiqNidec_A : Constant  Value=TRUE  OutDataTypeStr=boolean
  slr1_{1..28} (28 alike) : BusSelector  OutputSignals=VINP_CANMsgValidMCUNR1_flg
  slr_VHAL_MCUNR1CSErr_flg : BusSelector  OutputSignals=VHAL_MCUNR1CSErr_flg
  slr_VHAL_MCUNR1RCErr_flg : BusSelector  OutputSignals=VHAL_MCUNR1RCErr_flg
  slr_VHAL_MCUWarnRNidec_enum : BusSelector  OutputSignals=VHAL_MCUWarnRNidec_enum
  slr_VHAL_RrActvDmpDisabStaNidec_flg : BusSelector  OutputSignals=VHAL_RrActvDmpDisabStaNidec_flg
  slr_VHAL_RrEDUDrtStaNidec_flg : BusSelector  OutputSignals=VHAL_RrEDUDrtStaNidec_flg
  slr_VHAL_RrEDUOpratingStaNidec_flg : BusSelector  OutputSignals=VHAL_RrEDUOpratingStaNidec_flg
  slr_VHAL_RrEDURealTMTqNidec_Nm : BusSelector  OutputSignals=VHAL_RrEDURealTMTqNidec_Nm
  slr_VHAL_RrEDURotateDirctionNidec_enum : BusSelector  OutputSignals=VHAL_RrEDURotateDirctionNidec_enum
  slr_VHAL_RrEDUTqReqFbkNidec_Nm : BusSelector  OutputSignals=VHAL_RrEDUTqReqFbkNidec_Nm
  slr_VHAL_RrMCU1ChksumNidec_enum : BusSelector  OutputSignals=VHAL_RrMCU1ChksumNidec_enum
  slr_VHAL_RrMCU1RolCntNidec_enum : BusSelector  OutputSignals=VHAL_RrMCU1RolCntNidec_enum
  slr_VHAL_RrMCUBATNidec_V : BusSelector  OutputSignals=VHAL_RrMCUBATNidec_V
  slr_VHAL_RrMCUDCBusCurrNidec_A : BusSelector  OutputSignals=VHAL_RrMCUDCBusCurrNidec_A
  slr_VHAL_RrMCUDCBusVoltNidec_V : BusSelector  OutputSignals=VHAL_RrMCUDCBusVoltNidec_V
  slr_VHAL_RrMCUDischrgStaNidec_flg : BusSelector  OutputSignals=VHAL_RrMCUDischrgStaNidec_flg
  slr_VHAL_RrMCUEnaStaNidec_flg : BusSelector  OutputSignals=VHAL_RrMCUEnaStaNidec_flg
  slr_VHAL_RrMCUErrNidec_enum : BusSelector  OutputSignals=VHAL_RrMCUErrNidec_enum
  slr_VHAL_RrMCUIGNstaNidec_flg : BusSelector  OutputSignals=VHAL_RrMCUIGNstaNidec_flg
  slr_VHAL_RrMCUReady4PreNidec_flg : BusSelector  OutputSignals=VHAL_RrMCUReady4PreNidec_flg
  slr_VHAL_RrMCUReadyNidec_flg : BusSelector  OutputSignals=VHAL_RrMCUReadyNidec_flg
  slr_VHAL_RrMCUSysStaNidec_enum : BusSelector  OutputSignals=VHAL_RrMCUSysStaNidec_enum
  slr_VHAL_RrMCUTempNidec_C : BusSelector  OutputSignals=VHAL_RrMCUTempNidec_C
  slr_VHAL_RrMotorAvailTqNidec_Nm : BusSelector  OutputSignals=VHAL_RrMotorAvailTqNidec_Nm
  slr_VHAL_RrRegenAvailTqNidec_Nm : BusSelector  OutputSignals=VHAL_RrRegenAvailTqNidec_Nm
  slr_VHAL_RrTMSpdNidec_rpm : BusSelector  OutputSignals=VHAL_RrTMSpdNidec_rpm
  slr_VHAL_RrTMTempNidec_C : BusSelector  OutputSignals=VHAL_RrTMTempNidec_C
  slr_VHAL_RrTMidNidec_A : BusSelector  OutputSignals=VHAL_RrTMidNidec_A
  slr_VHAL_RrTMiqNidec_A : BusSelector  OutputSignals=VHAL_RrTMiqNidec_A
  VINP_MCUNR1CSErr_flg : Outport
  VINP_MCUNR1RCErr_flg : Outport  Port=2
  VINP_MCUWarnRNidec_enum : Outport  Port=3
  VINP_RrActvDmpDisabStaNidec_flg : Outport  Port=4
  VINP_RrEDUDrtStaNidec_flg : Outport  Port=5
  VINP_RrEDUOpratingStaNidec_flg : Outport  Port=6
  VINP_RrEDURealTMTqNidec_Nm : Outport  Port=7
  VINP_RrEDURotateDirctionNidec_enum : Outport  Port=8
  VINP_RrEDUTqReqFbkNidec_Nm : Outport  Port=9
  VINP_RrMCU1ChksumNidec_enum : Outport  Port=10
  VINP_RrMCU1RolCntNidec_enum : Outport  Port=11
  VINP_RrMCUBATNidec_V : Outport  Port=12
  VINP_RrMCUDCBusCurrNidec_A : Outport  Port=13
  VINP_RrMCUDCBusVoltNidec_V : Outport  Port=14
  VINP_RrMCUDischrgStaNidec_flg : Outport  Port=15
  VINP_RrMCUEnaStaNidec_flg : Outport  Port=16
  VINP_RrMCUErrNidec_enum : Outport  Port=17
  VINP_RrMCUIGNstaNidec_flg : Outport  Port=18
  VINP_RrMCUReady4PreNidec_flg : Outport  Port=19
  VINP_RrMCUReadyNidec_flg : Outport  Port=20
  VINP_RrMCUSysStaNidec_enum : Outport  Port=21
  VINP_RrMCUTempNidec_C : Outport  Port=22
  VINP_RrMotorAvailTqNidec_Nm : Outport  Port=23
  VINP_RrRegenAvailTqNidec_Nm : Outport  Port=24
  VINP_RrTMSpdNidec_rpm : Outport  Port=25
  VINP_RrTMTempNidec_C : Outport  Port=26
  VINP_RrTMidNidec_A : Outport  Port=27
  VINP_RrTMiqNidec_A : Outport  Port=28
  wires:
  BHAL_outputs/1 -> [BHAL_outputs]
  inp_CanValid_bus/1 -> [inp_CanValid_bus]
  [BHAL_outputs] -> slr_VHAL_MCUNR1CSErr_flg/1
  slr_VHAL_MCUNR1CSErr_flg/1 -> MCUNR1CSErr/1  "<VHAL_MCUNR1CSErr_flg>"
  True_VHAL_MCUNR1CSErr_flg/1 -> MCUNR1CSErr/2
  [inp_CanValid_bus] -> slr1_1/1
  slr1_1/1 -> MCUNR1CSErr/3  "<VINP_CANMsgValidMCUNR1_flg>"
  MCUNR1CSErr/1 -> VINP_MCUNR1CSErr_flg/1  "VINP_MCUNR1CSErr_flg"
  MCUNR1CSErr/2 -> Terminator_1/1
  [BHAL_outputs] -> slr_VHAL_MCUNR1RCErr_flg/1
  slr_VHAL_MCUNR1RCErr_flg/1 -> MCUNR1RCErr/1  "<VHAL_MCUNR1RCErr_flg>"
  True_VHAL_MCUNR1RCErr_flg/1 -> MCUNR1RCErr/2
  [inp_CanValid_bus] -> slr1_2/1
  slr1_2/1 -> MCUNR1RCErr/3  "<VINP_CANMsgValidMCUNR1_flg>"
  MCUNR1RCErr/1 -> VINP_MCUNR1RCErr_flg/1  "VINP_MCUNR1RCErr_flg"
  MCUNR1RCErr/2 -> Terminator_2/1
  [BHAL_outputs] -> slr_VHAL_MCUWarnRNidec_enum/1
  slr_VHAL_MCUWarnRNidec_enum/1 -> MCUWarnRNidec/1  "<VHAL_MCUWarnRNidec_enum>"
  True_VHAL_MCUWarnRNidec_enum/1 -> MCUWarnRNidec/2
  [inp_CanValid_bus] -> slr1_3/1
  slr1_3/1 -> MCUWarnRNidec/3  "<VINP_CANMsgValidMCUNR1_flg>"
  MCUWarnRNidec/1 -> VINP_MCUWarnRNidec_enum/1  "VINP_MCUWarnRNidec_enum"
  MCUWarnRNidec/2 -> Terminator_3/1
  [BHAL_outputs] -> slr_VHAL_RrActvDmpDisabStaNidec_flg/1
  slr_VHAL_RrActvDmpDisabStaNidec_flg/1 -> RrActvDmpDisabStaNidec/1  "<VHAL_RrActvDmpDisabStaNidec_flg>"
  True_VHAL_RrActvDmpDisabStaNidec_flg/1 -> RrActvDmpDisabStaNidec/2
  [inp_CanValid_bus] -> slr1_4/1
  slr1_4/1 -> RrActvDmpDisabStaNidec/3  "<VINP_CANMsgValidMCUNR1_flg>"
  RrActvDmpDisabStaNidec/1 -> VINP_RrActvDmpDisabStaNidec_flg/1  "VINP_RrActvDmpDisabStaNidec_flg"
  RrActvDmpDisabStaNidec/2 -> Terminator_4/1
  [BHAL_outputs] -> slr_VHAL_RrEDUDrtStaNidec_flg/1
  slr_VHAL_RrEDUDrtStaNidec_flg/1 -> RrEDUDrtStaNidec/1  "<VHAL_RrEDUDrtStaNidec_flg>"
  True_VHAL_RrEDUDrtStaNidec_flg/1 -> RrEDUDrtStaNidec/2
  [inp_CanValid_bus] -> slr1_5/1
  slr1_5/1 -> RrEDUDrtStaNidec/3  "<VINP_CANMsgValidMCUNR1_flg>"
  RrEDUDrtStaNidec/1 -> VINP_RrEDUDrtStaNidec_flg/1  "VINP_RrEDUDrtStaNidec_flg"
  RrEDUDrtStaNidec/2 -> Terminator_5/1
  [BHAL_outputs] -> slr_VHAL_RrEDUOpratingStaNidec_flg/1
  slr_VHAL_RrEDUOpratingStaNidec_flg/1 -> RrEDUOpratingStaNidec/1  "<VHAL_RrEDUOpratingStaNidec_flg>"
  True_VHAL_RrEDUOpratingStaNidec_flg/1 -> RrEDUOpratingStaNidec/2
  [inp_CanValid_bus] -> slr1_6/1
  slr1_6/1 -> RrEDUOpratingStaNidec/3  "<VINP_CANMsgValidMCUNR1_flg>"
  RrEDUOpratingStaNidec/1 -> VINP_RrEDUOpratingStaNidec_flg/1  "VINP_RrEDUOpratingStaNidec_flg"
  RrEDUOpratingStaNidec/2 -> Terminator_6/1
  [BHAL_outputs] -> slr_VHAL_RrEDURealTMTqNidec_Nm/1
  slr_VHAL_RrEDURealTMTqNidec_Nm/1 -> RrEDURealTMTqNidec/1  "<VHAL_RrEDURealTMTqNidec_Nm>"
  True_VHAL_RrEDURealTMTqNidec_Nm/1 -> RrEDURealTMTqNidec/2
  [inp_CanValid_bus] -> slr1_7/1
  slr1_7/1 -> RrEDURealTMTqNidec/3  "<VINP_CANMsgValidMCUNR1_flg>"
  RrEDURealTMTqNidec/1 -> VINP_RrEDURealTMTqNidec_Nm/1  "VINP_RrEDURealTMTqNidec_Nm"
  RrEDURealTMTqNidec/2 -> Terminator_7/1
  [BHAL_outputs] -> slr_VHAL_RrEDURotateDirctionNidec_enum/1
  slr_VHAL_RrEDURotateDirctionNidec_enum/1 -> RrEDURotateDirctionNidec/1  "<VHAL_RrEDURotateDirctionNidec_enum>"
  True_VHAL_RrEDURotateDirctionNidec_enum/1 -> RrEDURotateDirctionNidec/2
  [inp_CanValid_bus] -> slr1_8/1
  slr1_8/1 -> RrEDURotateDirctionNidec/3  "<VINP_CANMsgValidMCUNR1_flg>"
  RrEDURotateDirctionNidec/1 -> VINP_RrEDURotateDirctionNidec_enum/1  "VINP_RrEDURotateDirctionNidec_enum"
  RrEDURotateDirctionNidec/2 -> Terminator_8/1
  [BHAL_outputs] -> slr_VHAL_RrEDUTqReqFbkNidec_Nm/1
  slr_VHAL_RrEDUTqReqFbkNidec_Nm/1 -> RrEDUTqReqFbkNidec/1  "<VHAL_RrEDUTqReqFbkNidec_Nm>"
  True_VHAL_RrEDUTqReqFbkNidec_Nm/1 -> RrEDUTqReqFbkNidec/2
  [inp_CanValid_bus] -> slr1_9/1
  slr1_9/1 -> RrEDUTqReqFbkNidec/3  "<VINP_CANMsgValidMCUNR1_flg>"
  RrEDUTqReqFbkNidec/1 -> VINP_RrEDUTqReqFbkNidec_Nm/1  "VINP_RrEDUTqReqFbkNidec_Nm"
  RrEDUTqReqFbkNidec/2 -> Terminator_9/1
  [BHAL_outputs] -> slr_VHAL_RrMCU1ChksumNidec_enum/1
  slr_VHAL_RrMCU1ChksumNidec_enum/1 -> RrMCU1ChksumNidec/1  "<VHAL_RrMCU1ChksumNidec_enum>"
  True_VHAL_RrMCU1ChksumNidec_enum/1 -> RrMCU1ChksumNidec/2
  [inp_CanValid_bus] -> slr1_10/1
  slr1_10/1 -> RrMCU1ChksumNidec/3  "<VINP_CANMsgValidMCUNR1_flg>"
  RrMCU1ChksumNidec/1 -> VINP_RrMCU1ChksumNidec_enum/1  "VINP_RrMCU1ChksumNidec_enum"
  RrMCU1ChksumNidec/2 -> Terminator_10/1
  [BHAL_outputs] -> slr_VHAL_RrMCU1RolCntNidec_enum/1
  slr_VHAL_RrMCU1RolCntNidec_enum/1 -> RrMCU1RolCntNidec/1  "<VHAL_RrMCU1RolCntNidec_enum>"
  True_VHAL_RrMCU1RolCntNidec_enum/1 -> RrMCU1RolCntNidec/2
  [inp_CanValid_bus] -> slr1_11/1
  slr1_11/1 -> RrMCU1RolCntNidec/3  "<VINP_CANMsgValidMCUNR1_flg>"
  RrMCU1RolCntNidec/1 -> VINP_RrMCU1RolCntNidec_enum/1  "VINP_RrMCU1RolCntNidec_enum"
  RrMCU1RolCntNidec/2 -> Terminator_11/1
  [BHAL_outputs] -> slr_VHAL_RrMCUBATNidec_V/1
  slr_VHAL_RrMCUBATNidec_V/1 -> RrMCUBATNidec/1  "<VHAL_RrMCUBATNidec_V>"
  True_VHAL_RrMCUBATNidec_V/1 -> RrMCUBATNidec/2
  [inp_CanValid_bus] -> slr1_12/1
  slr1_12/1 -> RrMCUBATNidec/3  "<VINP_CANMsgValidMCUNR1_flg>"
  RrMCUBATNidec/1 -> VINP_RrMCUBATNidec_V/1  "VINP_RrMCUBATNidec_V"
  RrMCUBATNidec/2 -> Terminator_12/1
  [BHAL_outputs] -> slr_VHAL_RrMCUDCBusCurrNidec_A/1
  slr_VHAL_RrMCUDCBusCurrNidec_A/1 -> RrMCUDCBusCurrNidec/1  "<VHAL_RrMCUDCBusCurrNidec_A>"
  True_VHAL_RrMCUDCBusCurrNidec_A/1 -> RrMCUDCBusCurrNidec/2
  [inp_CanValid_bus] -> slr1_13/1
  slr1_13/1 -> RrMCUDCBusCurrNidec/3  "<VINP_CANMsgValidMCUNR1_flg>"
  RrMCUDCBusCurrNidec/1 -> VINP_RrMCUDCBusCurrNidec_A/1  "VINP_RrMCUDCBusCurrNidec_A"
  RrMCUDCBusCurrNidec/2 -> Terminator_13/1
  [BHAL_outputs] -> slr_VHAL_RrMCUDCBusVoltNidec_V/1
  slr_VHAL_RrMCUDCBusVoltNidec_V/1 -> RrMCUDCBusVoltNidec/1  "<VHAL_RrMCUDCBusVoltNidec_V>"
  True_VHAL_RrMCUDCBusVoltNidec_V/1 -> RrMCUDCBusVoltNidec/2
  [inp_CanValid_bus] -> slr1_14/1
  slr1_14/1 -> RrMCUDCBusVoltNidec/3  "<VINP_CANMsgValidMCUNR1_flg>"
  RrMCUDCBusVoltNidec/1 -> VINP_RrMCUDCBusVoltNidec_V/1  "VINP_RrMCUDCBusVoltNidec_V"
  RrMCUDCBusVoltNidec/2 -> Terminator_14/1
  [BHAL_outputs] -> slr_VHAL_RrMCUDischrgStaNidec_flg/1
  slr_VHAL_RrMCUDischrgStaNidec_flg/1 -> RrMCUDischrgStaNidec/1  "<VHAL_RrMCUDischrgStaNidec_flg>"
  True_VHAL_RrMCUDischrgStaNidec_flg/1 -> RrMCUDischrgStaNidec/2
  [inp_CanValid_bus] -> slr1_15/1
  slr1_15/1 -> RrMCUDischrgStaNidec/3  "<VINP_CANMsgValidMCUNR1_flg>"
  RrMCUDischrgStaNidec/1 -> VINP_RrMCUDischrgStaNidec_flg/1  "VINP_RrMCUDischrgStaNidec_flg"
  RrMCUDischrgStaNidec/2 -> Terminator_15/1
  [BHAL_outputs] -> slr_VHAL_RrMCUEnaStaNidec_flg/1
  slr_VHAL_RrMCUEnaStaNidec_flg/1 -> RrMCUEnaStaNidec/1  "<VHAL_RrMCUEnaStaNidec_flg>"
  True_VHAL_RrMCUEnaStaNidec_flg/1 -> RrMCUEnaStaNidec/2
  [inp_CanValid_bus] -> slr1_16/1
  slr1_16/1 -> RrMCUEnaStaNidec/3  "<VINP_CANMsgValidMCUNR1_flg>"
  RrMCUEnaStaNidec/1 -> VINP_RrMCUEnaStaNidec_flg/1  "VINP_RrMCUEnaStaNidec_flg"
  RrMCUEnaStaNidec/2 -> Terminator_16/1
  [BHAL_outputs] -> slr_VHAL_RrMCUErrNidec_enum/1
  slr_VHAL_RrMCUErrNidec_enum/1 -> RrMCUErrNidec/1  "<VHAL_RrMCUErrNidec_enum>"
  True_VHAL_RrMCUErrNidec_enum/1 -> RrMCUErrNidec/2
  [inp_CanValid_bus] -> slr1_17/1
  slr1_17/1 -> RrMCUErrNidec/3  "<VINP_CANMsgValidMCUNR1_flg>"
  RrMCUErrNidec/1 -> VINP_RrMCUErrNidec_enum/1  "VINP_RrMCUErrNidec_enum"
  RrMCUErrNidec/2 -> Terminator_17/1
  [BHAL_outputs] -> slr_VHAL_RrMCUIGNstaNidec_flg/1
  slr_VHAL_RrMCUIGNstaNidec_flg/1 -> RrMCUIGNstaNidec/1  "<VHAL_RrMCUIGNstaNidec_flg>"
  True_VHAL_RrMCUIGNstaNidec_flg/1 -> RrMCUIGNstaNidec/2
  [inp_CanValid_bus] -> slr1_18/1
  slr1_18/1 -> RrMCUIGNstaNidec/3  "<VINP_CANMsgValidMCUNR1_flg>"
  RrMCUIGNstaNidec/1 -> VINP_RrMCUIGNstaNidec_flg/1  "VINP_RrMCUIGNstaNidec_flg"
  RrMCUIGNstaNidec/2 -> Terminator_18/1
  [BHAL_outputs] -> slr_VHAL_RrMCUReady4PreNidec_flg/1
  slr_VHAL_RrMCUReady4PreNidec_flg/1 -> RrMCUReady4PreNidec/1  "<VHAL_RrMCUReady4PreNidec_flg>"
  True_VHAL_RrMCUReady4PreNidec_flg/1 -> RrMCUReady4PreNidec/2
  [inp_CanValid_bus] -> slr1_19/1
  slr1_19/1 -> RrMCUReady4PreNidec/3  "<VINP_CANMsgValidMCUNR1_flg>"
  RrMCUReady4PreNidec/1 -> VINP_RrMCUReady4PreNidec_flg/1  "VINP_RrMCUReady4PreNidec_flg"
  RrMCUReady4PreNidec/2 -> Terminator_19/1
  [BHAL_outputs] -> slr_VHAL_RrMCUReadyNidec_flg/1
  slr_VHAL_RrMCUReadyNidec_flg/1 -> RrMCUReadyNidec/1  "<VHAL_RrMCUReadyNidec_flg>"
  True_VHAL_RrMCUReadyNidec_flg/1 -> RrMCUReadyNidec/2
  [inp_CanValid_bus] -> slr1_20/1
  slr1_20/1 -> RrMCUReadyNidec/3  "<VINP_CANMsgValidMCUNR1_flg>"
  RrMCUReadyNidec/1 -> VINP_RrMCUReadyNidec_flg/1  "VINP_RrMCUReadyNidec_flg"
  RrMCUReadyNidec/2 -> Terminator_20/1
  [BHAL_outputs] -> slr_VHAL_RrMCUSysStaNidec_enum/1
  slr_VHAL_RrMCUSysStaNidec_enum/1 -> RrMCUSysStaNidec/1  "<VHAL_RrMCUSysStaNidec_enum>"
  True_VHAL_RrMCUSysStaNidec_enum/1 -> RrMCUSysStaNidec/2
  [inp_CanValid_bus] -> slr1_21/1
  slr1_21/1 -> RrMCUSysStaNidec/3  "<VINP_CANMsgValidMCUNR1_flg>"
  RrMCUSysStaNidec/1 -> VINP_RrMCUSysStaNidec_enum/1  "VINP_RrMCUSysStaNidec_enum"
  RrMCUSysStaNidec/2 -> Terminator_21/1
  [BHAL_outputs] -> slr_VHAL_RrMCUTempNidec_C/1
  slr_VHAL_RrMCUTempNidec_C/1 -> RrMCUTempNidec/1  "<VHAL_RrMCUTempNidec_C>"
  True_VHAL_RrMCUTempNidec_C/1 -> RrMCUTempNidec/2
  [inp_CanValid_bus] -> slr1_22/1
  slr1_22/1 -> RrMCUTempNidec/3  "<VINP_CANMsgValidMCUNR1_flg>"
  RrMCUTempNidec/1 -> VINP_RrMCUTempNidec_C/1  "VINP_RrMCUTempNidec_C"
  RrMCUTempNidec/2 -> Terminator_22/1
  [BHAL_outputs] -> slr_VHAL_RrMotorAvailTqNidec_Nm/1
  slr_VHAL_RrMotorAvailTqNidec_Nm/1 -> RrMotorAvailTqNidec/1  "<VHAL_RrMotorAvailTqNidec_Nm>"
  True_VHAL_RrMotorAvailTqNidec_Nm/1 -> RrMotorAvailTqNidec/2
  [inp_CanValid_bus] -> slr1_23/1
  slr1_23/1 -> RrMotorAvailTqNidec/3  "<VINP_CANMsgValidMCUNR1_flg>"
  RrMotorAvailTqNidec/1 -> VINP_RrMotorAvailTqNidec_Nm/1  "VINP_RrMotorAvailTqNidec_Nm"
  RrMotorAvailTqNidec/2 -> Terminator_23/1
  [BHAL_outputs] -> slr_VHAL_RrRegenAvailTqNidec_Nm/1
  slr_VHAL_RrRegenAvailTqNidec_Nm/1 -> RrRegenAvailTqNidec/1  "<VHAL_RrRegenAvailTqNidec_Nm>"
  True_VHAL_RrRegenAvailTqNidec_Nm/1 -> RrRegenAvailTqNidec/2
  [inp_CanValid_bus] -> slr1_24/1
  slr1_24/1 -> RrRegenAvailTqNidec/3  "<VINP_CANMsgValidMCUNR1_flg>"
  RrRegenAvailTqNidec/1 -> VINP_RrRegenAvailTqNidec_Nm/1  "VINP_RrRegenAvailTqNidec_Nm"
  RrRegenAvailTqNidec/2 -> Terminator_24/1
  [BHAL_outputs] -> slr_VHAL_RrTMSpdNidec_rpm/1
  slr_VHAL_RrTMSpdNidec_rpm/1 -> RrTMSpdNidec/1  "<VHAL_RrTMSpdNidec_rpm>"
  True_VHAL_RrTMSpdNidec_rpm/1 -> RrTMSpdNidec/2
  [inp_CanValid_bus] -> slr1_25/1
  slr1_25/1 -> RrTMSpdNidec/3  "<VINP_CANMsgValidMCUNR1_flg>"
  RrTMSpdNidec/1 -> VINP_RrTMSpdNidec_rpm/1  "VINP_RrTMSpdNidec_rpm"
  RrTMSpdNidec/2 -> Terminator_25/1
  [BHAL_outputs] -> slr_VHAL_RrTMTempNidec_C/1
  slr_VHAL_RrTMTempNidec_C/1 -> RrTMTempNidec/1  "<VHAL_RrTMTempNidec_C>"
  True_VHAL_RrTMTempNidec_C/1 -> RrTMTempNidec/2
  [inp_CanValid_bus] -> slr1_26/1
  slr1_26/1 -> RrTMTempNidec/3  "<VINP_CANMsgValidMCUNR1_flg>"
  RrTMTempNidec/1 -> VINP_RrTMTempNidec_C/1  "VINP_RrTMTempNidec_C"
  RrTMTempNidec/2 -> Terminator_26/1
  [BHAL_outputs] -> slr_VHAL_RrTMidNidec_A/1
  slr_VHAL_RrTMidNidec_A/1 -> RrTMidNidec/1  "<VHAL_RrTMidNidec_A>"
  True_VHAL_RrTMidNidec_A/1 -> RrTMidNidec/2
  [inp_CanValid_bus] -> slr1_27/1
  slr1_27/1 -> RrTMidNidec/3  "<VINP_CANMsgValidMCUNR1_flg>"
  RrTMidNidec/1 -> VINP_RrTMidNidec_A/1  "VINP_RrTMidNidec_A"
  RrTMidNidec/2 -> Terminator_27/1
  [BHAL_outputs] -> slr_VHAL_RrTMiqNidec_A/1
  slr_VHAL_RrTMiqNidec_A/1 -> RrTMiqNidec/1  "<VHAL_RrTMiqNidec_A>"
  True_VHAL_RrTMiqNidec_A/1 -> RrTMiqNidec/2
  [inp_CanValid_bus] -> slr1_28/1
  slr1_28/1 -> RrTMiqNidec/3  "<VINP_CANMsgValidMCUNR1_flg>"
  RrTMiqNidec/1 -> VINP_RrTMiqNidec_A/1  "VINP_RrTMiqNidec_A"
  RrTMiqNidec/2 -> Terminator_28/1
